simulink model "chap7_2sim"  (Simulink 7.0)
settings: Solver=ode45  StartTime=0.0  StopTime=30  FixedStep=0.001  RelTol=1e-3
settings Model: Creator=Administrator  LastModifiedBy=eleliuj  ExtModeTrigMode=oneshot  ExtModeArmWhenConnect=off
settings DataIOCC: LimitDataPoints=off  SignalLoggingName=sigsOut
settings OptimizationCC: BooleanDataType=off
settings DebuggingCC: SaveWithParameterizedLinksMsg=none  SignalResolutionControl=TryResolveAllWithWarning  SolverPrmCheckMsg=none  MultiTaskDSMMsg=warning  MultiTaskCondExecSysMsg=none  StrictBusMsg=None
settings HardwareCC: TargetUnknown=on
settings RTWCC: IncludeERTFirstTime=on

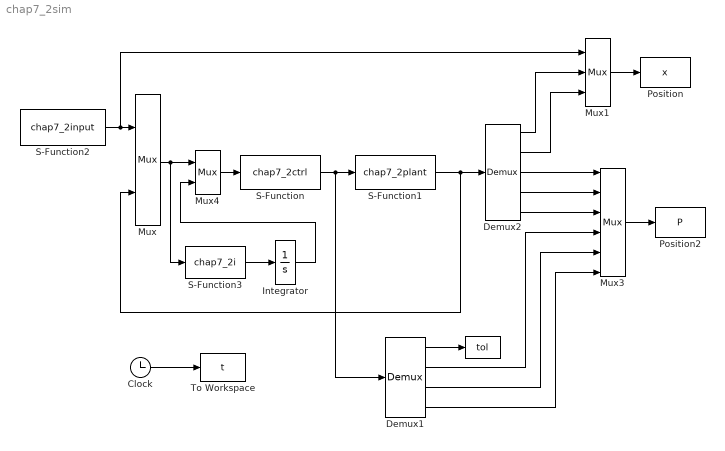
== system chap7_2sim ==
  " " : ToWorkspace  VariableName=tol  SampleTime=-1  SaveFormat=Array
  Clock : Clock
      settings: Decimation=10
  Demux1 : Demux
  Demux2 : Demux  Outputs=5
  Integrator : Integrator
  Mux : Mux  Inputs=2
  Mux1 : Mux  Inputs=3
  Mux3 : Mux  Inputs=6
  Mux4 : Mux  Inputs=2
  Position : ToWorkspace  VariableName=x  SampleTime=-1  SaveFormat=Array
  Position2 : ToWorkspace  VariableName=P  SampleTime=-1  SaveFormat=Array
  S-Function : S-Function  FunctionName=chap7_2ctrl
  S-Function1 : S-Function  FunctionName=chap7_2plant
  S-Function2 : S-Function  FunctionName=chap7_2input
  S-Function3 : S-Function  FunctionName=chap7_2i
  To Workspace : ToWorkspace  VariableName=t  SampleTime=-1  SaveFormat=Array
  wires:
  Mux/1 -> S-Function3/1, Mux4/1
  Demux2/1 -> Mux1/2
  S-Function1/1 -> Demux2/1, Mux/2
  S-Function2/1 -> Mux/1, Mux1/1
  Demux1/1 -> " "/1
  Mux1/1 -> Position/1
  S-Function/1 -> S-Function1/1, Demux1/1
  Mux3/1 -> Position2/1
  Mux4/1 -> S-Function/1
  S-Function3/1 -> Integrator/1
  Integrator/1 -> Mux4/2
  Clock/1 -> To Workspace/1
  Demux2/2 -> Mux1/3
  Demux2/3 -> Mux3/1
  Demux2/4 -> Mux3/2
  Demux2/5 -> Mux3/3
  Demux1/2 -> Mux3/4
  Demux1/3 -> Mux3/5
  Demux1/4 -> Mux3/6
